simulink model "psbtriphaseline"  (Simulink 6.0)
settings: Solver=ode15s  SolverMode=SingleTasking  StartTime=0.0  StopTime=0.1  RelTol=1e-3  AbsTol=1e-6
libraries: powerlib2 x23
settings Model: Creator=patrice  LastModifiedBy=batserve  ExtModeTrigMode=oneshot  ExtModeArmWhenConnect=off  ExtModeAutoUpdateStatusClock=off
settings DataIOCC: LimitDataPoints=off  SignalLoggingName=sigsOut
settings OptimizationCC: BlockReduction=off  BooleanDataType=off
settings DebuggingCC: CheckExecutionContextPreStartOutputMsg=on  CheckExecutionContextRuntimeOutputMsg=on  SolverPrmCheckMsg=none  IntegerOverflowMsg=none
settings HardwareCC: TargetUnknown=on
settings RTWCC: TemplateMakefile=grt_unix.tmf

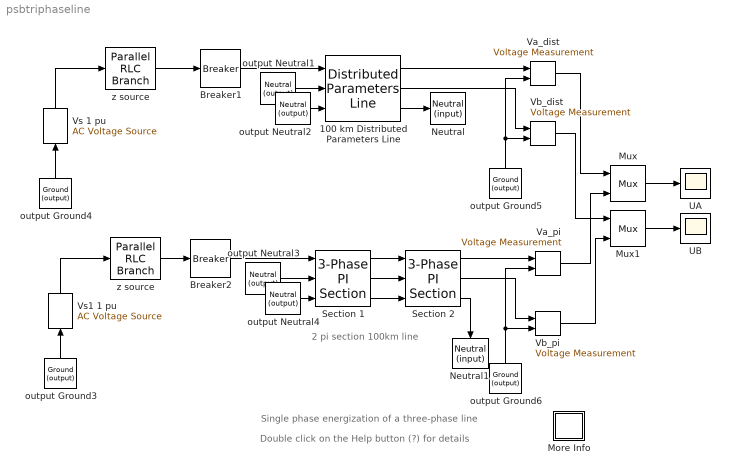
== system psbtriphaseline ==
  note: Double click on the Help button (?) for details
  note: 2 pi section 100km line
  note: Single phase energization of a three-phase line
  100 km Distributed Parameters Line : powerlib2/Elements/Distributed Parameters Line  Tag=PoWeRsYsTeMbLoCk  n=3  f=60  r=[0.01273 0.3864]  l="[0.9337e-3  4.1264e-3]"  c=[12.74e-9 7.751e-9]  lgt=100  x1=[0 0 0 0; 0.0001244 0 0 0; 0.0002488 0 0 0; 0.0003733 0 0 0; 0.0004977 0 0 0; 0.0006221 0 0 0]  x2=[0 0 0 0; 0.0001244 0 0 0; 0.0002488 0 0 0; 0.0003733 0 0 0; 0.0004977 0 0 0; 0.0006221 0 0 0]  x3=[0 0 0 0; 0.0001244 0 0 0; 0.0002488 0 0 0; 0.0003733 0 0 0; 0.0004977 0 0 0; 0.0006221 0 0 0]  x4=[0 0 0 0; 0.0001244 0 0 0; 0.0002488 0 0 0; 0.0003733 0 0 0; 0.0004977 0 0 0; 0.0006221 0 0 0]  x5=0  mesure=None  PSBOutputType=111111111111111111111111111111
  Breaker1 : powerlib2/Elements/Breaker  Tag=PoWeRsYsTeMbLoCk  a=0.01  c=0  rs=inf  cs=0  times="[ 0.25/60  4/60 ]"  Ts=0  comext=off  mesure=None  PSBOutputType=1
  Breaker2 : powerlib2/Elements/Breaker  Tag=PoWeRsYsTeMbLoCk  a=0.01  c=0  rs=inf  cs=0  times="[ .25/60  4/60 ]"  Ts=0  comext=off  mesure=None  PSBOutputType=1
  More Info : Subsystem
      mask Display: disp('?')
  Mux : Mux  Inputs=2
  Mux1 : Mux  Inputs=2
  Neutral : powerlib2/Connectors/Neutral (input)  Tag=PoWeRsYsTeMbLoCk  no=995
  Neutral1 : powerlib2/Connectors/Neutral (input)  Tag=PoWeRsYsTeMbLoCk  Orientation=down  no=996
  Section 1 : powerlib2/Elements/3-Phase PI Section  f=60  R10=[ 0.01273 0.3864]  L10="[ 0.9337e-3  4.1264e-3]"  C10=[12.74e-9 7.751e-9]  long=50
  Section 2 : powerlib2/Elements/3-Phase PI Section  f=60  R10=[ 0.01273 0.3864]  L10="[ 0.9337e-3  4.1264e-3]"  C10=[12.74e-9 7.751e-9]  long=50
  UA : Scope
      settings: TickLabels=on  TimeRange=0.1  YMin=-4  YMax=4  DataFormat=Array
  UB : Scope
      settings: TickLabels=on  TimeRange=0.1  YMin=-1  YMax=1  DataFormat=Array  MaxDataPoints=500000
  Va_dist : powerlib2/Measurements/Voltage Measurement  Tag=PoWeRsYsTeMmEaSuReMeNt  PhasorSimulation=off  OutputType=Magnitude  PSBOutputType=0  PSBequivalent=0
  Va_pi : powerlib2/Measurements/Voltage Measurement  Tag=PoWeRsYsTeMmEaSuReMeNt  PhasorSimulation=off  OutputType=Magnitude  PSBOutputType=0  PSBequivalent=0
  Vb_dist : powerlib2/Measurements/Voltage Measurement  Tag=PoWeRsYsTeMmEaSuReMeNt  PhasorSimulation=off  OutputType=Magnitude  PSBOutputType=0  PSBequivalent=0
  Vb_pi : powerlib2/Measurements/Voltage Measurement  Tag=PoWeRsYsTeMmEaSuReMeNt  PhasorSimulation=off  OutputType=Magnitude  PSBOutputType=0  PSBequivalent=0
  Vs 1 pu : powerlib2/Electrical Sources/AC Voltage Source  Tag=PoWeRsYsTeMbLoCk  Orientation=up  A=1  P=0  F=60  stime=0  mesure=None  PSBOutputType=1
  Vs1 1 pu : powerlib2/Electrical Sources/AC Voltage Source  Tag=PoWeRsYsTeMbLoCk  Orientation=up  A=1  P=0  F=60  stime=0  mesure=None  PSBOutputType=1
  output Ground{3..6} (4 alike) : powerlib2/Connectors/Ground (output)  Tag=PoWeRsYsTeMbLoCk  Orientation=up  PSBOutputType=1
  output Neutral1 : powerlib2/Connectors/Neutral (output)  Tag=PoWeRsYsTeMbLoCk  no=991  PSBOutputType=1
  output Neutral2 : powerlib2/Connectors/Neutral (output)  Tag=PoWeRsYsTeMbLoCk  no=992  PSBOutputType=1
  output Neutral3 : powerlib2/Connectors/Neutral (output)  Tag=PoWeRsYsTeMbLoCk  no=993  PSBOutputType=1
  output Neutral4 : powerlib2/Connectors/Neutral (output)  Tag=PoWeRsYsTeMbLoCk  no=994  PSBOutputType=1
  z source : powerlib2/Elements/Parallel RLC Branch  Tag=PoWeRsYsTeMbLoCk  a=180  b=47.8e-3  c=0  mesure=None  PSBOutputType=1
  "z source " : powerlib2/Elements/Parallel RLC Branch  Tag=PoWeRsYsTeMbLoCk  a=180  b=47.8e-3  c=0  mesure=None  PSBOutputType=1
  wires:
  Section 2/3 -> Neutral1/1
  100 km Distributed Parameters Line/3 -> Neutral/1
  output Neutral4/1 -> Section 1/3
  output Neutral3/1 -> Section 1/2
  output Neutral2/1 -> 100 km Distributed Parameters Line/3
  output Neutral1/1 -> 100 km Distributed Parameters Line/2
  Vb_dist/1 -> Mux1/1
  Va_dist/1 -> Mux/1
  100 km Distributed Parameters Line/1 -> Va_dist/1
  100 km Distributed Parameters Line/2 -> Vb_dist/1
  output Ground5/1 -> Vb_dist/2, Va_dist/2
  Breaker1/1 -> 100 km Distributed Parameters Line/1
  output Ground6/1 -> Va_pi/2, Vb_pi/2
  Section 2/2 -> Vb_pi/1
  Section 2/1 -> Va_pi/1
  Vb_pi/1 -> Mux1/2
  Mux1/1 -> UB/1
  Va_pi/1 -> Mux/2
  Section 1/3 -> Section 2/3
  Section 1/2 -> Section 2/2
  Section 1/1 -> Section 2/1
  Breaker2/1 -> Section 1/1
  "z source "/1 -> Breaker2/1
  Mux/1 -> UA/1
  z source/1 -> Breaker1/1
  output Ground4/1 -> Vs 1 pu/1
  Vs 1 pu/1 -> z source/1
  output Ground3/1 -> Vs1 1 pu/1
  Vs1 1 pu/1 -> "z source "/1

== system psbtriphaseline/More Info ==
  note: A 100 km, 3-phase line is energized on a 735 kV, 30 000 MVA  equivalent network.
      | The line is first energized on phase A at t = 1/4 cycle (maximum of source voltage) and then deenergized at t = 4 cycles.
      | Phase B and phase C are left open.
      | Switchings are performed simultaneously on two different line models:
      |
      | - Distributed parameter line
      | - 3-phase  PI section line consisting of two 50 km sections.
      |   (The three-phase PI Line Section  block is available in the 'Extras/Three-Phase' library.)
      |
      | Voltages obtained on phases A and B at the line receiving end with the two models are compared.
  note: This demonstration compares transients obtained with
      | a distributed parameter line model and a PI section line model
  note: Circuit Description
  note: Demonstration
  note: G. Sybille (Hydro-Quebec)
  note: Open the two scopes and start the simulation.
      | Compare the voltages obtained on phase A and  phase B (induced voltage) with the two models.
      | Zoom on voltages rigth after energizing and notice the sharp edges obtained with the distributed parameter line (yellow trace).
      | These voltage steps which are due to travelling wave reflections at both ends  of the line are filtered by the PI model.
      | Notice also that phases A and B stay charged at peak voltage when the breakers are opened.
